simulink model "lateral_dyn_constrained"  (R2020b)
settings: Solver=VariableStepAuto  StartTime=0.0  StopTime=10.0  RelTol=1e-3
model workspace (MAT data in the model file):
  Mass = 0
settings Model: ParameterArgumentNames=Mass  OrderedModelArguments=off  Creator=User  LastModifiedBy=Matthew

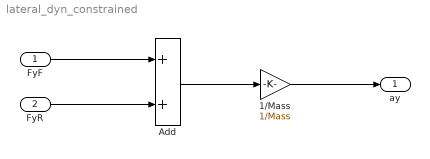
== system lateral_dyn_constrained ==
  FyF : Inport
  FyR : Inport  Port=2
  1/Mass : Gain  Gain=1/Mass
  Add : Sum
  ay : Outport
  wires:
  FyF/1 -> Add/1
  Add/1 -> 1/Mass/1
  1/Mass/1 -> ay/1
  FyR/1 -> Add/2
